simulink library "libMdl_TrainFrontDataGenerator"  (R2018a)
settings: Solver=VariableStepAuto  StartTime=0.0  StopTime=10.0  RelTol=1e-3
undefined symbols (not defined in the file): x_0
settings Model: Creator=hwinter  LastModifiedBy=Hanno

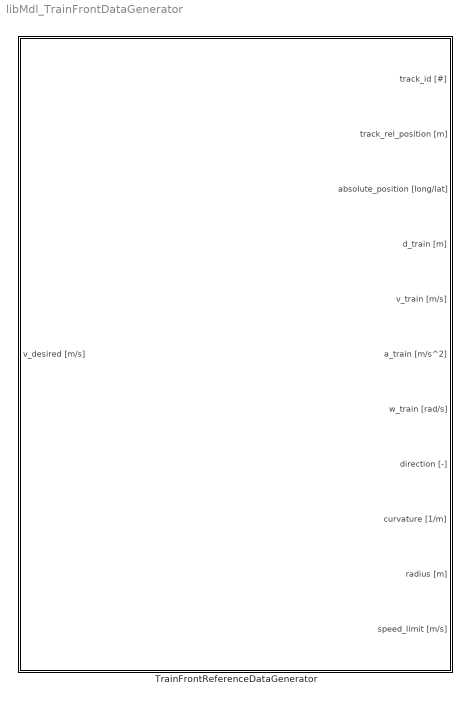
== system libMdl_TrainFrontDataGenerator ==
  TrainFrontReferenceDataGenerator : Subsystem  TreatAsAtomicUnit=on  SystemSampleTime=mv_T_ref_system  mask(Reference Data Generator (train front)){mv_T_ref_system=-1, mv_motion_t_constant=[], mv_a_train_limits=[], mv_track_id_0=[], mv_track_rel_position_0=[], mv_x_0=[], mv_track_map=[], mv_track_map_rot_angle=[]}
      mask prompts: mv_T_ref_system "Sample Time:"; mv_motion_t_constant "Motion Time Constant:"; mv_a_train_limits "Max Acceleration:"; mv_track_id_0 "Initial Track ID:"; mv_track_rel_position_0 "Initial distance:"; mv_x_0 "Initial v and a:"; mv_track_map "Track Map:"; mv_track_map_rot_angle "Track Map Rotation Angle:"
      mask help:
      | Sample Time:
      | Sample time of the block in seconds
      |
      | Motion Time Constant:
      | Time constant of the speed controller loop in seconds
      |
      | Max Acceleration:
      | Maximum acceleration with which the train is accelerated
      | (format: [max_neg_acc, max_pos_acc])
      |
      | Initial Track ID:
      | ID of the track, where the train starts
      |
      | Initial distance:
      | Distance in meters on the initial track, where the train starts
      |
      | Initial v and a:
      | Initial speed and acceleration
      | (format: [speed_0, acceleration_0])
      |
      | Track Map:
      | Track-Map in matrix format
      | (for more details see: Track Generator Tool)
      |
      | Track Map Rotation Angle:
      | Initial alignment of the Track-Map in degrees
      mask Display:
      | str1 = sprintf('\\color{black}{\\bfReference Data Generator (train front)}\n\n');
      | str2 = sprintf('Sample Time: %0.2f\n\n',mv_T_ref_system);
      | str3 = sprintf('Motion Time Constant: %0.2f\n',mv_motion_t_constant);
      | if length(mv_a_train_limits) > 1
      |     str4 = sprintf('a_{max}: %0.2f\n',mv_a_train_limits(2));
      |     str5 = sprintf('a_{min}: %0.2f\n\n',mv_a_train_limits(1));
      | else
      |     str4 = sprintf('a_{max}: %0.2f\n',mv_a_train_limits);
      |     str5 = sprintf('a_{min}: %0.2f\n',mv_a_train_limits);
      | end % if
      | str6 = sprintf('Initial Track ID: %i\n',mv_track_id_0);
      | str7 = sprintf('Initial distance: %0.2f\n',mv_track_rel_position_0);
      | if length(mv_x_0) <= 3
      |     str8 = sprintf('[v_0, a_0]: %s\n\n',mat2str(mv_x_0,5));
      | else
      |     str8 = sprintf('[v_0, a_0]: [...]\n\n');
      | end % if
      | if length(mv_track_map) == 1
      |     str9 = sprintf('Map: %0.2f\n',mv_track_map);
      | else
      |     str9 = sprintf('Map: [...]\n');
      | end % if
      | str10 = sprintf('\\phi_{Map}: %5.1f',mv_track_map_rot_angle);
      | str = [str1,str2,str3,str4,str5,str6,str7,str8,str9,str10];
      | 
      | text( 0.5,0.5, ...
      |       str, ...
      |       'horizontalAlignment', 'center', ...
      |       'texmode','on' ...
      |     )

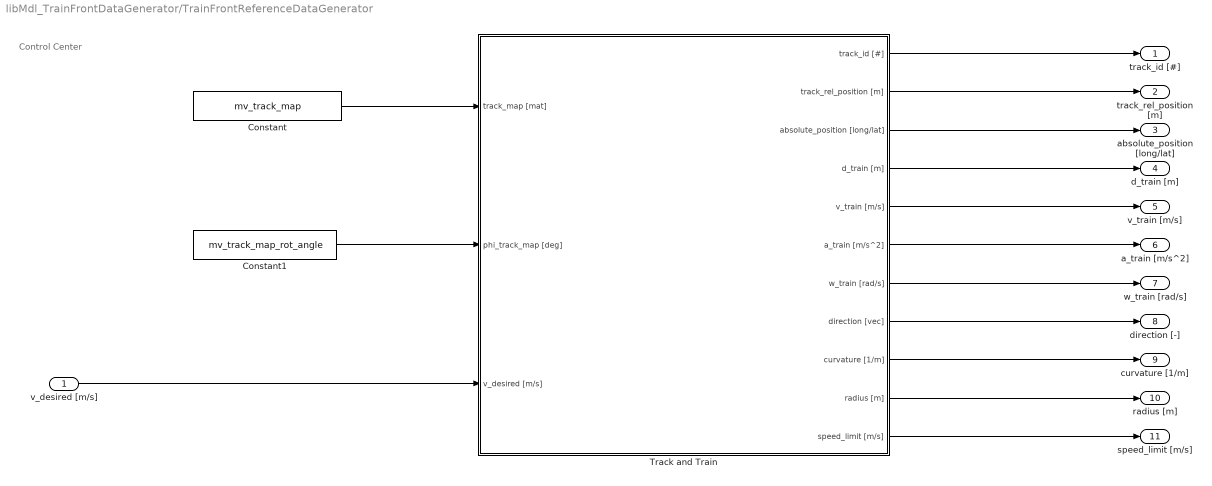
== system libMdl_TrainFrontDataGenerator/TrainFrontReferenceDataGenerator ==
  note: Control Center
  v_desired [m/s] : Inport
  Constant : Constant  Value=mv_track_map  VectorParams1D=off
  Constant1 : Constant  Value=mv_track_map_rot_angle
  Track and Train : Subsystem
  track_id [#] : Outport
  track_rel_position [m] : Outport  Port=2
  absolute_position [long/lat] : Outport  Port=3
  d_train [m] : Outport  Port=4
  v_train [m/s] : Outport  Port=5
  a_train [m/s^2] : Outport  Port=6
  w_train [rad/s] : Outport  Port=7
  direction [-] : Outport  Port=8
  curvature [1/m] : Outport  Port=9
  radius [m] : Outport  Port=10
  speed_limit [m/s] : Outport  Port=11
  wires:
  Constant1/1 -> Track and Train/2(phi_track_map [deg])
  Constant/1 -> Track and Train/1(track_map [mat])
  v_desired [m/s]/1 -> Track and Train/3(v_desired [m/s])
  Track and Train/7(w_train [rad/s]) -> w_train [rad/s]/1
  Track and Train/6(a_train [m/s^2]) -> a_train [m/s^2]/1
  Track and Train/5(v_train [m/s]) -> v_train [m/s]/1
  Track and Train/4(d_train [m]) -> d_train [m]/1
  Track and Train/10(radius [m]) -> radius [m]/1
  Track and Train/11(speed_limit [m/s]) -> speed_limit [m/s]/1
  Track and Train/9(curvature [1/m]) -> curvature [1/m]/1
  Track and Train/8(direction [vec]) -> direction [-]/1
  Track and Train/3(absolute_position [long/lat]) -> absolute_position [long/lat]/1
  Track and Train/2(track_rel_position [m]) -> track_rel_position [m]/1
  Track and Train/1(track_id [#]) -> track_id [#]/1

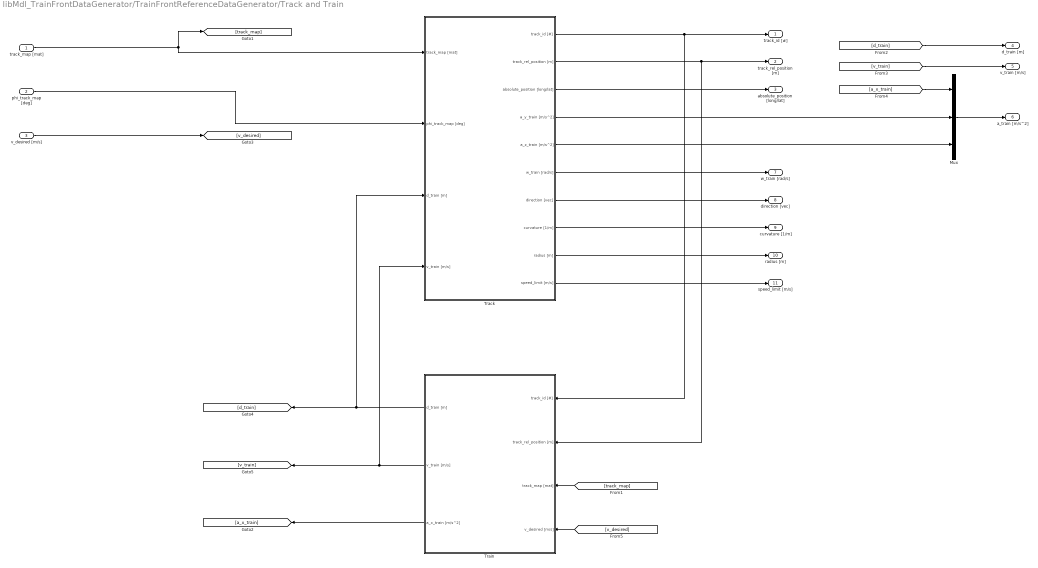
== system libMdl_TrainFrontDataGenerator/TrainFrontReferenceDataGenerator/Track and Train ==
  track_map [mat] : Inport
  phi_track_map [deg] : Inport  Port=2
  v_desired [m/s] : Inport  Port=3
  Mux : Mux  Inputs=3
  Track : Subsystem
  Train : Subsystem
  track_id [#] : Outport
  track_rel_position [m] : Outport  Port=2
  absolute_position [long/lat] : Outport  Port=3
  d_train [m] : Outport  Port=4
  v_train [m/s] : Outport  Port=5
  a_train [m/s^2] : Outport  Port=6
  w_train [rad/s] : Outport  Port=7
  direction [vec] : Outport  Port=8
  curvature [1/m] : Outport  Port=9
  radius [m] : Outport  Port=10
  speed_limit [m/s] : Outport  Port=11
  wires:
  Track/7(direction [vec]) -> direction [vec]/1
  Track/8(curvature [1/m]) -> curvature [1/m]/1
  Track/9(radius [m]) -> radius [m]/1
  Track/10(speed_limit [m/s]) -> speed_limit [m/s]/1
  Track/6(w_train [rad/s]) -> w_train [rad/s]/1
  Track/3(absolute_position [long/lat]) -> absolute_position [long/lat]/1
  Track/2(track_rel_position [m]) -> Train/2(track_rel_position [m]), track_rel_position [m]/1
  Track/1(track_id [#]) -> Train/1(track_id [#]), track_id [#]/1
  [v_train] -> v_train [m/s]/1
  [d_train] -> d_train [m]/1
  Train/2(v_train [m/s]) -> [v_train], Track/4(v_train [m/s])
  Train/3(a_x_train [m/s^2]) -> [a_x_train]
  [v_desired] -> Train/4(v_desired [m/s])
  phi_track_map [deg]/1 -> Track/2(phi_track_map [deg])
  track_map [mat]/1 -> Track/1(track_map [mat]), [track_map]
  v_desired [m/s]/1 -> [v_desired]
  [track_map] -> Train/3(track_map [mat])
  Train/1(d_train [m]) -> Track/3(d_train [m]), [d_train]
  Track/4(a_y_train [m/s^2]) -> Mux/2
  Track/5(a_z_train [m/s^2]) -> Mux/3
  [a_x_train] -> Mux/1
  Mux/1 -> a_train [m/s^2]/1

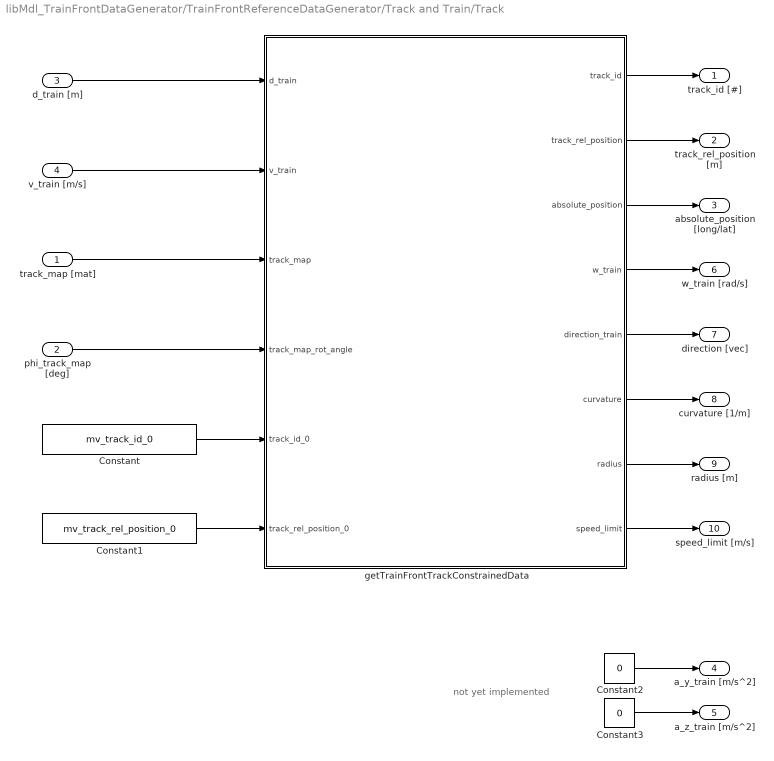
== system libMdl_TrainFrontDataGenerator/TrainFrontReferenceDataGenerator/Track and Train/Track ==
  note: not yet implemented
  track_map [mat] : Inport
  phi_track_map [deg] : Inport  Port=2
  d_train [m] : Inport  Port=3
  v_train [m/s] : Inport  Port=4
  Constant : Constant  Value=mv_track_id_0
  Constant1 : Constant  Value=mv_track_rel_position_0
  Constant2 : Constant  Value=0
  Constant3 : Constant  Value=0
  getTrainFrontTrackConstrainedData : MATLAB Function  TreatAsAtomicUnit=on
  track_id [#] : Outport
  track_rel_position [m] : Outport  Port=2
  absolute_position [long/lat] : Outport  Port=3
  a_y_train [m/s^2] : Outport  Port=4
  a_z_train [m/s^2] : Outport  Port=5
  w_train [rad/s] : Outport  Port=6
  direction [vec] : Outport  Port=7
  curvature [1/m] : Outport  Port=8
  radius [m] : Outport  Port=9
  speed_limit [m/s] : Outport  Port=10
  wires:
  Constant1/1 -> getTrainFrontTrackConstrainedData/6(track_rel_position_0)
  Constant/1 -> getTrainFrontTrackConstrainedData/5(track_id_0)
  getTrainFrontTrackConstrainedData/8(speed_limit) -> speed_limit [m/s]/1
  getTrainFrontTrackConstrainedData/7(radius) -> radius [m]/1
  getTrainFrontTrackConstrainedData/6(curvature) -> curvature [1/m]/1
  getTrainFrontTrackConstrainedData/5(direction_train) -> direction [vec]/1
  getTrainFrontTrackConstrainedData/4(w_train) -> w_train [rad/s]/1
  getTrainFrontTrackConstrainedData/3(absolute_position) -> absolute_position [long/lat]/1
  getTrainFrontTrackConstrainedData/2(track_rel_position) -> track_rel_position [m]/1
  getTrainFrontTrackConstrainedData/1(track_id) -> track_id [#]/1
  phi_track_map [deg]/1 -> getTrainFrontTrackConstrainedData/4(track_map_rot_angle)
  v_train [m/s]/1 -> getTrainFrontTrackConstrainedData/2(v_train)
  track_map [mat]/1 -> getTrainFrontTrackConstrainedData/3(track_map)
  d_train [m]/1 -> getTrainFrontTrackConstrainedData/1(d_train)
  Constant2/1 -> a_y_train [m/s^2]/1
  Constant3/1 -> a_z_train [m/s^2]/1

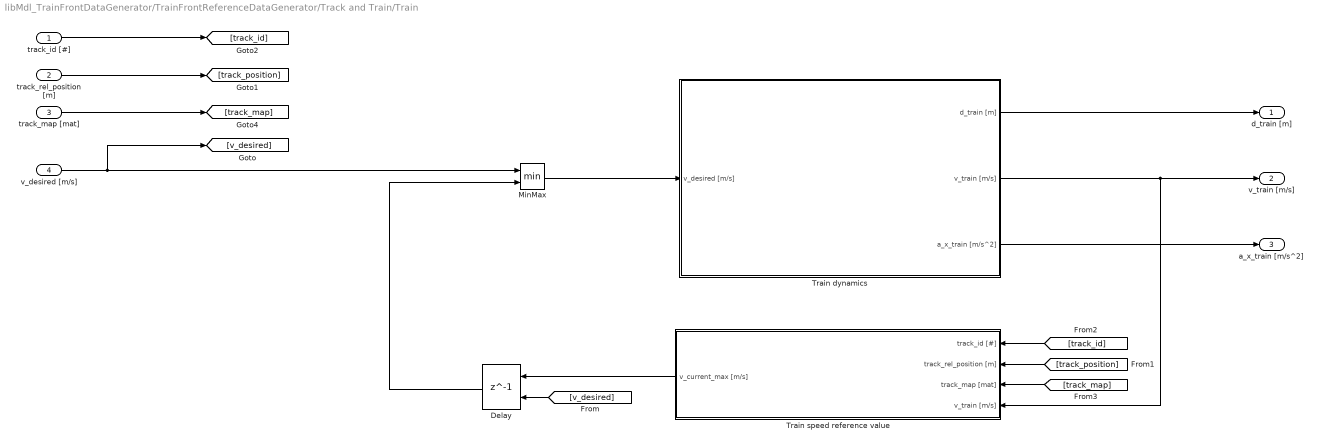
== system libMdl_TrainFrontDataGenerator/TrainFrontReferenceDataGenerator/Track and Train/Train ==
  track_id [#] : Inport
  track_rel_position [m] : Inport  Port=2
  track_map [mat] : Inport  Port=3
  v_desired [m/s] : Inport  Port=4
  Delay : Delay  DelayLength=1  InitialConditionSource=Input port  InitialCondition=x_0
      settings: InputPortMap=u0,p4
  MinMax : MinMax  Inputs=2
  Train dynamics : Subsystem  TreatAsAtomicUnit=on
  Train speed reference value : Subsystem  TreatAsAtomicUnit=on
  d_train [m] : Outport
  v_train [m/s] : Outport  Port=2
  a_x_train [m/s^2] : Outport  Port=3
  wires:
  MinMax/1 -> Train dynamics/1(v_desired [m/s])
  Delay/1 -> MinMax/2
  Train speed reference value/1(v_current_max [m/s]) -> Delay/1
  [track_id] -> Train speed reference value/1(track_id [#])
  track_id [#]/1 -> [track_id]
  [track_map] -> Train speed reference value/3(track_map [mat])
  track_map [mat]/1 -> [track_map]
  track_rel_position [m]/1 -> [track_position]
  Train dynamics/3(a_x_train [m/s^2]) -> a_x_train [m/s^2]/1
  Train dynamics/1(d_train [m]) -> d_train [m]/1
  Train dynamics/2(v_train [m/s]) -> Train speed reference value/4(v_train [m/s]), v_train [m/s]/1
  [v_desired] -> Delay/2
  v_desired [m/s]/1 -> [v_desired], MinMax/1
  [track_position] -> Train speed reference value/2(track_rel_position [m])

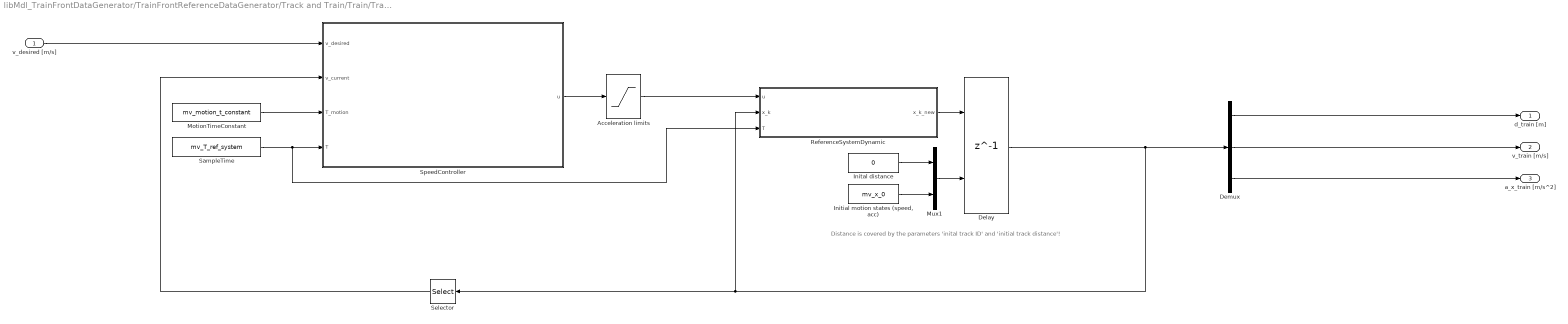
== system libMdl_TrainFrontDataGenerator/TrainFrontReferenceDataGenerator/Track and Train/Train/Train dynamics ==
  note: Distance is covered by the parameters 'inital track ID' and 'initial track distance'!
  v_desired [m/s] : Inport
  Acceleration limits : Saturate  UpperLimit=mv_a_train_limits(2)  LowerLimit=mv_a_train_limits(1)
  Delay : Delay  DelayLength=1  InitialConditionSource=Input port  InitialCondition=x_0
      settings: InputPortMap=u0,p4
  Demux : Demux  Outputs=3
  Inital distance : Constant  Value=0
  "Initial motion states (speed, acc)" : Constant  Value=mv_x_0
  MotionTimeConstant : Constant  Value=mv_motion_t_constant
  Mux1 : Mux  Inputs=2
  ReferenceSystemDynamic : MATLAB Function  TreatAsAtomicUnit=on
  SampleTime : Constant  Value=mv_T_ref_system
  Selector : Selector  InputPortWidth=3  IndexOptions=Index vector (dialog)  Indices=2  OutputSizes=1
  SpeedController : MATLAB Function  TreatAsAtomicUnit=on
  d_train [m] : Outport
  v_train [m/s] : Outport  Port=2
  a_x_train [m/s^2] : Outport  Port=3
  wires:
  Acceleration limits/1 -> ReferenceSystemDynamic/1(u)
  ReferenceSystemDynamic/1(x_k_new) -> Delay/1
  Mux1/1 -> Delay/2
  Delay/1 -> Demux/1, ReferenceSystemDynamic/2(x_k), Selector/1
  "Initial motion states (speed, acc)"/1 -> Mux1/2
  Inital distance/1 -> Mux1/1
  Demux/3 -> a_x_train [m/s^2]/1
  Demux/2 -> v_train [m/s]/1
  Demux/1 -> d_train [m]/1
  v_desired [m/s]/1 -> SpeedController/1(v_desired)
  Selector/1 -> SpeedController/2(v_current)
  SpeedController/1(u) -> Acceleration limits/1
  SampleTime/1 -> SpeedController/4(T), ReferenceSystemDynamic/3(T)
  MotionTimeConstant/1 -> SpeedController/3(T_motion)

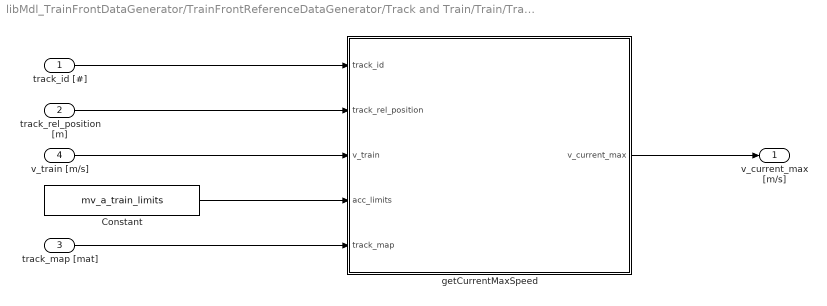
== system libMdl_TrainFrontDataGenerator/TrainFrontReferenceDataGenerator/Track and Train/Train/Train speed reference value ==
  track_id [#] : Inport
  track_rel_position [m] : Inport  Port=2
  track_map [mat] : Inport  Port=3
  v_train [m/s] : Inport  Port=4
  Constant : Constant  Value=mv_a_train_limits
  getCurrentMaxSpeed : MATLAB Function  TreatAsAtomicUnit=on
  v_current_max [m/s] : Outport
  wires:
  track_id [#]/1 -> getCurrentMaxSpeed/1(track_id)
  Constant/1 -> getCurrentMaxSpeed/4(acc_limits)
  getCurrentMaxSpeed/1(v_current_max) -> v_current_max [m/s]/1
  v_train [m/s]/1 -> getCurrentMaxSpeed/3(v_train)
  track_rel_position [m]/1 -> getCurrentMaxSpeed/2(track_rel_position)
  track_map [mat]/1 -> getCurrentMaxSpeed/5(track_map)

== matlab function libMdl_TrainFrontDataGenerator/TrainFrontReferenceDataGenerator/Track and Train/Track/getTrainFrontTrackConstrainedData ==
  data: d_train input; v_train input; track_id output; track_rel_position output; absolute_position output; w_train output; direction_train output; track_map input; curvature output; track_map_rot_angle input; radius output; speed_limit output; track_id_0 input; track_rel_position_0 input
function [track_id,track_rel_position,absolute_position,w_train,direction_train,curvature,radius,speed_limit] = simFcn_getTrainFrontTrackConstrainedData(d_train,v_train,track_map,track_map_rot_angle,track_id_0,track_rel_position_0)

% Init ____________________________________________________________________

coder.extrinsic('calcTrackProperties');

track_id = coder.nullcopy(zeros(1,1));
track_rel_position = coder.nullcopy(zeros(1,1));
absolute_position = coder.nullcopy(zeros(2,1));
w_train = coder.nullcopy(zeros(3,1));
direction_train = coder.nullcopy(zeros(2,1));
curvature = coder.nullcopy(zeros(1,1));
radius = coder.nullcopy(zeros(1,1));
speed_limit = coder.nullcopy(zeros(1,1));

% Calculations ____________________________________________________________

% set direction of train on the track
track_direction = sign(d_train);
track_direction(track_direction==0) = sign(v_train);
track_direction(track_direction==0) = 1;

% calculate output values
[track_id,track_rel_position,~,absolute_position,direction_train,curvature,radius,speed_limit] = calcTrackProperties(d_train,track_id_0,track_rel_position_0,track_map,track_map_rot_angle,track_direction);

w_train = [0;0;-1*curvature*v_train]; % roll rate not implemented yet 
                                        % pitch rate not implemented yet
                                        % yaw rate: multiply by minus 1 to transform from track coordinates (curvature) to train coordinates (turn rate)
speed_limit = speed_limit/3.6; % transform km/h to m/s

end

== matlab function libMdl_TrainFrontDataGenerator/TrainFrontReferenceDataGenerator/Track and Train/Train/Train speed reference value/getCurrentMaxSpeed ==
  data: track_id input; track_rel_position input; v_train input; acc_limits input; track_map input; v_current_max output
function v_current_max = simFcn_getCurrentMaxSpeed(track_id,track_rel_position,v_train,acc_limits,track_map)

coder.extrinsic('calcCurrentMaxSpeed');
v_current_max = coder.nullcopy(zeros(1));

v_current_max = calcCurrentMaxSpeed(track_id,track_rel_position,acc_limits,v_train,track_map);

end

== matlab function libMdl_TrainFrontDataGenerator/TrainFrontReferenceDataGenerator/Track and Train/Train/Train dynamics/SpeedController ==
  data: v_desired input; v_current input; T_motion input; u output; T input
function u = simFcn_SpeedController(v_desired,v_current,T_motion,T)

% System
A = 1; b = T; c = 1;

% Desired poles (in z-plane)
% T_controller = (v_desired/(100/3.6)*mv_controller_t_constant/5);
T_controller = T_motion;
p_desired = exp(T*(-1/T_controller));

% Calculate controller (see appended calculations at the bottom)
k = -(p_desired - 1)/T;
prefilter = (c'*(eye(length(A))-A+b*k')^-1*b)^-1;

% Controller output
u = prefilter*v_desired - k'*v_current;

end % function speedController

%% Notes

% syms s k1 p1 T
% 
% A = [1];
% b = [T];
% k = [k1];
% 
% p = [p1];
% 
% Ak = A - b*k.';
% 
% Pist = collect(simplify(det([s*eye(length(Ak)) - Ak])),s);
% Psoll = collect(simplify((s-p(1))),s);
% 
% a_i = coeffs(Pist,s,'All');
% a_i_soll = coeffs(Psoll,s,'All');
% 
% [k1_final] = solve([a_i_soll==a_i],[k1]);
% 
% k1_final = simplify(k1_final)

== matlab function libMdl_TrainFrontDataGenerator/TrainFrontReferenceDataGenerator/Track and Train/Train/Train dynamics/ReferenceSystemDynamic ==
  data: u input; x_k_new output; x_k input; T input
function x_k_new  = simFcn_ReferenceSystemDynamic(u,x_k,T)
% x_k_new  = simFcn_ReferenceSystemDynamic(x_k,T)
%
% x_k = [distance, speed, acceleration]'

F = [ 1   T   0; ... 
      0   1   0; ...
      0   0   0];
x_k_new = F*x_k + [1/2*T^2;T;1]*u;

end % function
